simulink model "mconversion10"  (Simulink 6.0)
settings: Solver=ode3  StartTime=0.0  StopTime=10.0  RelTol=1e-3
settings Model: Creator=awarlock  LastModifiedBy=awarlock  ExtModeAutoUpdateStatusClock=off
settings OptimizationCC: InlineParams=on
settings DebuggingCC: CheckExecutionContextPreStartOutputMsg=on  CheckExecutionContextRuntimeOutputMsg=on  SolverPrmCheckMsg=none  InheritedTsInSrcMsg=none
settings SFSimCC: SFSimApplyToAllLibs=on  SFSimBuildMode=Incremental

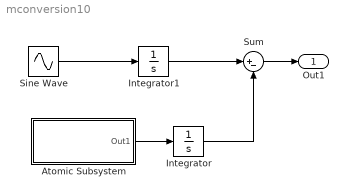
== system mconversion10 ==
  Atomic Subsystem : Subsystem  TreatAsAtomicUnit=on  PropExecContextAcrossSSBoundary=on
  Integrator : Integrator
  Integrator1 : Integrator
  Sine Wave : Sin  SampleTime=0
  Sum : Sum  Inputs=|+-
  Out1 : Outport
  wires:
  Sum/1 -> Out1/1
  Sine Wave/1 -> Integrator1/1
  Atomic Subsystem/1(Out1) -> Integrator/1
  Integrator/1 -> Sum/2
  Integrator1/1 -> Sum/1

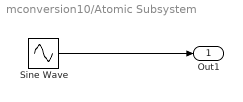
== system mconversion10/Atomic Subsystem ==
  Sine Wave : Sin
  Out1 : Outport
  wires:
  Sine Wave/1 -> Out1/1
